simulink subsystem "MC_CAN"  (R2023b)
settings: Solver=VariableStepAuto  StartTime=0.0  StopTime=10.0  RelTol=1e-3
settings Model: Creator=diego  LastModifiedBy=diego

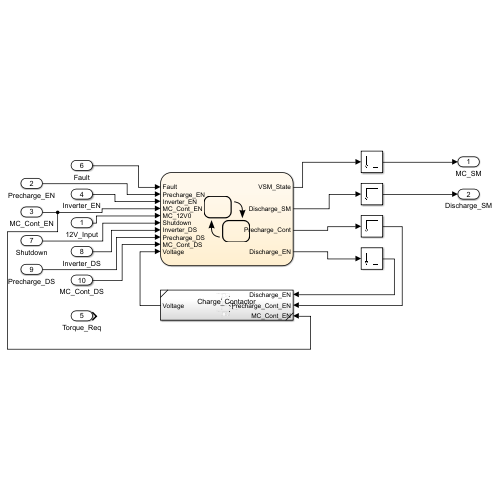
[thumbnail: Simulink's stored preview of the top-level diagram]
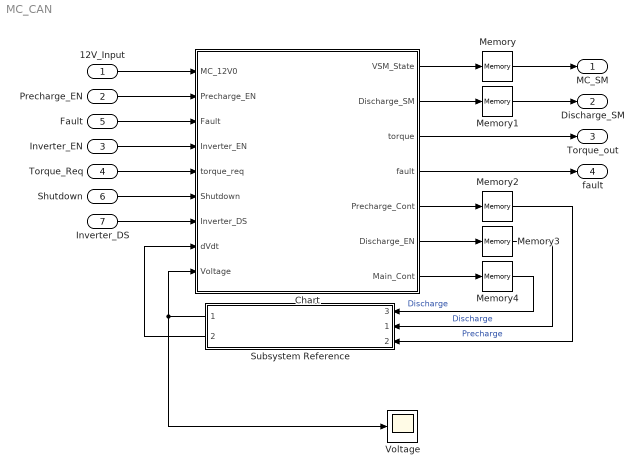
== system MC_CAN ==
  12V_Input : Inport
  Precharge_EN : Inport  Port=2
  Inverter_EN : Inport  Port=3
  Torque_Req : Inport  Port=4
  Fault : Inport  Port=5
  Shutdown : Inport  Port=6
  Inverter_DS : Inport  Port=7
  Chart : Stateflow chart  TreatAsAtomicUnit=on
      settings: PortSchema="{\"entries\":[{\"content\":{\"sides\":[{\"content\":{\"connectorIds\":[\"In4\",\"In2\",\"In1\",\"In3\",\"In8\",\"In5\",\"In7\",\"In9\",\"In6\"]},\"type\":\"ConnectorPlacement.EquallySpacedRectSide\",\"uuid\":\"03599179-c40e-45c0-8f83-03707e7643a9\"},{\"content\":{\"connectorIds\":[\"Out1\",\"Out2\",\"Out6\",\"Out7\",\"Out3\",\"Out4\",\"Out5\"],\"side\":\"RIGHT\"},\"type\":\"ConnectorPlacement.EquallySpacedRectSide\",\"uuid\":\"77c27c81-6b7f-49bb-b8ad-65b312eda7e2\"},{\"content\":{\"side\":\"TOP\"},\"type\":\"ConnectorPlacement.EquallySpacedRectSide\",\"uuid\":\"12a0a04d-7874-431f-b4d8-e9223037e866\"}]},\"type\":\"ConnectorPlacement.EquallySpacedConnector\",\"uuid\":\"58e614a8-4325-4fa7-852b-761998465240\"}],\"packageUris\":[\"http://schema.mathworks.com/mf0/Connector/R2020b\"],\"version\":\"1.0\"}"
  Memory{,1..4} (5 alike) : Memory
  Subsystem Reference : Subsystem  ReferencedSubsystem=Charge_Contactor
      settings: PortSchema="{\"entries\":[{\"content\":{\"sides\":[{\"content\":{\"connectorIds\":[\"In3\",\"In1\",\"In2\"]},\"type\":\"ConnectorPlacement.EquallySpacedRectSide\",\"uuid\":\"c4a26b2a-75b7-46e9-83ad-f08a209eb654\"},{\"content\":{\"connectorIds\":[\"Out1\",\"Out2\"],\"side\":\"RIGHT\"},\"type\":\"ConnectorPlacement.EquallySpacedRectSide\",\"uuid\":\"e0e23db8-3606-4757-a6fd-db7c1d3e8c5a\"},{\"content\":{\"side\":\"TOP\"},\"type\":\"ConnectorPlacement.EquallySpacedRectSide\",\"uuid\":\"0a967cd1-2252-4813-adc7-d3e8433b462a\"}]},\"type\":\"ConnectorPlacement.EquallySpacedConnector\",\"uuid\":\"d4c2dd3c-9ab6-4575-a91c-d1aa35d96284\"}],\"packageUris\":[\"http://schema.mathworks.com/mf0/Connector/R2020b\"],\"version\":\"1.0\"}"
  Voltage : Scope
  MC_SM : Outport
  Discharge_SM : Outport  Port=2
  Torque_out : Outport  Port=3
  fault : Outport  Port=4
  wires:
  Chart/2(Discharge_SM) -> Memory1/1
  Chart/3(Precharge_Cont) -> Memory2/1
  Fault/1 -> Chart/1(Fault)
  Subsystem Reference/1 -> Chart/6(Voltage), Voltage/1
  Memory1/1 -> Discharge_SM/1
  Inverter_EN/1 -> Chart/3(Inverter_EN)
  Memory/1 -> MC_SM/1
  Precharge_EN/1 -> Chart/2(Precharge_EN)
  Inverter_DS/1 -> Chart/7(Inverter_DS)
  12V_Input/1 -> Chart/4(MC_12V0)
  Chart/1(VSM_State) -> Memory/1
  Shutdown/1 -> Chart/5(Shutdown)
  Chart/4(Discharge_EN) -> Memory3/1
  Memory3/1 -> Subsystem Reference/1  "Discharge"
  Memory2/1 -> Subsystem Reference/2  "Precharge"
  Torque_Req/1 -> Chart/8(torque_req)
  Chart/6(torque) -> Torque_out/1
  Subsystem Reference/2 -> Chart/9(dVdt)
  Chart/5(Main_Cont) -> Memory4/1
  Memory4/1 -> Subsystem Reference/3  "Discharge"
  Chart/7(fault) -> fault/1

== stateflow chart MC_CAN/Chart ==
  state Motor_Controller
    state Start
      entry:
      VSM_State = 0;
    state Precharge
      entry:
      VSM_State = 1;
      dV = 1000;
      state Precharge2
        entry:
        VSM_State = 3;
        dV = dVdt
      state Precharge3
        entry:
        VSM_State = 4;
        Precharge_Cont = 0;
        Main_Cont = 1;
      state Precharge1
        entry:
        VSM_State = 2;
        Precharge_Cont = 1;
      (default) -> Precharge1
      Precharge1 -> Precharge2
      Precharge2 -> Precharge3 : [dV<56]
    state Fault
      entry:
      VSM_State = 9;
      state Fault_ON
        fault =1;
      state Fault_OFF
        fault = 0;
      (default) -> Fault_ON
      Fault_ON -> Fault_OFF : after(Pulse, sec)
    state Running
      entry:
      VSM_State = 6;
      during:
      torque = torque_req;
      exit:
      torque = 0;
    state Ready
      entry:
      VSM_State = 5;
    state Shutdown
      entry:
      VSM_State = 14;
      Discharge_SM = 0;
      Discharge_EN = 0;
    state Discharge
      entry:
      VSM_State = 7;
      Main_Cont = 0;
      state Discharge1
        entry:
        Discharge_SM = 1;
        Discharge_EN = 1;
      state Discharge2
        entry:
        Discharge_SM = 2;
      state Discharge4
        entry:
        Discharge_SM = 4;
      state Discharge3
        entry:
        Discharge_SM = 3;
      (default) -> Discharge1
      Discharge1 -> Discharge2
      Discharge2 -> Discharge3 : [RPM < 75]
      Discharge3 -> Discharge4 : [ Voltage < 30]
    (default) -> Start
    Shutdown -> Start : [MC_12V0 == 0]
    Start -> Precharge : [Precharge_EN == 1]
    Precharge3 -> Ready
    Motor_Controller -> Fault [order 2] : [Fault ==1 && fault ~= 1 && Discharge_EN ~= 1]
    Fault_OFF -> Discharge : [MC_12V0 == 0]
    Ready -> Running : [Inverter_EN == 1]
    Running -> Ready : [Inverter_DS == 1]
    Discharge -> Shutdown : [Discharge_SM == 4]
    Motor_Controller -> Discharge [order 1] : [Shutdown == 1]
  (default) -> Motor_Controller
  data: Fault input; VSM_State output [0..14] =0; Precharge_EN input; Inverter_EN input; Discharge_SM output =1; RPM local =0; MC_12V0 input; Shutdown input; Precharge_Cont output; Voltage input =0; Inverter_DS input; Discharge_EN output =0; Main_Cont output =0; torque_req input; torque output; dVdt input; dV local; Pulse local =.2; fault output =0
